simulink model "WT_FINAL_PERFECT_FIT"  (R2025a)
settings: Solver=ode4  StartTime=0.0  StopTime=11  FixedStep=0.1  RelTol=1e-3
libraries: simulink x1
settings Model: Creator=hero  LastModifiedBy=hero

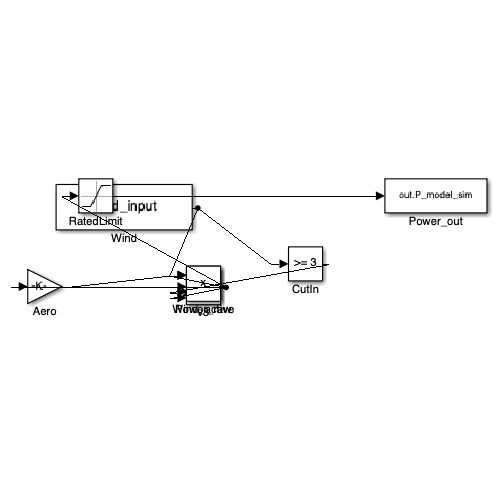
[thumbnail: Simulink's stored preview of the top-level diagram]
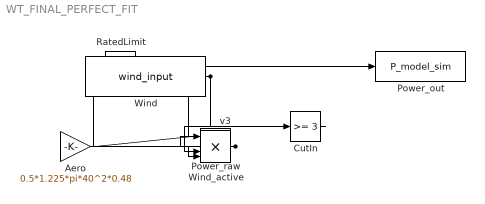
== system WT_FINAL_PERFECT_FIT ==
  Aero : Gain  Gain=0.5*1.225*pi*40^2*0.48
  CutIn : simulink/Logic and Bit Operations/Compare To Constant  relop=>=  const=3  OutDataTypeStr=boolean
  Power_out : ToWorkspace  VariableName=P_model_sim  SampleTime=-1
  Power_raw : Product
  RatedLimit : Saturate  UpperLimit=652.7945  LowerLimit=0
  Wind : FromWorkspace  VariableName=wind_input
  Wind_active : Product
  v3 : Product  Inputs=3
  wires:
  Wind/1 -> CutIn/1, Wind_active/1
  CutIn/1 -> Wind_active/2
  Wind_active/1 -> v3/1, v3/2, v3/3
  v3/1 -> Aero/1
  Aero/1 -> Power_raw/1
  Power_raw/1 -> RatedLimit/1
  RatedLimit/1 -> Power_out/1
